simulink library "EngineSystemSubmodel"  (R2014b)
settings: Solver=ode45  StartTime=0.0  StopTime=10.0  FixedStep=1e-4  RelTol=1e-3
values from neighbouring files (symbols this model uses):
  D_turb_wheel = TC.TC_map.turb.D_wheel    [init_MVM.m]
  delta = 2    [Init8RTFLEX68D.m]    (also in Untitled2.m = fcn(p); fcn.m = zeros(size(p)))
  eta_turb_max = TC.TC_map.turb.eff_max    [init_MVM.m]
  flow_coeff_turb = [-1.585326540339;-4.823836967181;1.5853156139822]    [Init8RTFLEX68D.m]    (also in init_MVM.m = TC.TC_map.turb.flow_fit_coeff)
  fs = 0.0683    [Init8RTFLEX68D.m]    (also in NOxProcessGUI.m = varargin{2}; initHybrid.m; initMV.m; init_MVM.m = 0.0682925799315)
  genset = generators(1)    [runTempCyl4S.m]
  J_tc = TC.SAE_map_comp.inertia    [init_MVM.m]
  kai = 1.7    [Init8RTFLEX68D.m]
  Kb = 1*ones(engines,1)    [initHybrid.m]    (also in initMV.m; init_MVM.m = 1; init_ele.m = 1)
  Kd = 20*ones(engines,1)    [initHybrid.m]    (also in initMV.m; init_MVM.m = 10; init_ele.m = 20)
  Ki = 20*ones(engines,1)    [initHybrid.m]    (also in initMV.m; init_MVM.m = 10; init_ele.m = 20)
  Kp = 20*ones(engines,1)    [initHybrid.m]    (also in initMV.m; init_MVM.m = 10; init_ele.m = 20)
  Load_amp = x(4) + xRef(i)    [GetErrGensetResp.m]    (also in runsimulation.m = 0.55; runsimulationRecovery.m = InitialLoad(jj) + LoadStep(ii))
  Load_bias = x(4)    [GetErrGensetResp.m]    (also in runsimulation.m = 0.15; runsimulationRecovery.m = InitialLoad(jj))
  Load_index = 1    [GetErrGensetResp.m]    (also in runsimulation.m; runsimulationRecovery.m)
  N = x*noMol    [NOxProcessGUI.m]    (also in initHybrid.m = .1*ones(engines,1); initMV.m = .1*ones(engines,1); init_ele.m = 0.1)
  omegat0 = RPM_TC_initial/30*pi    [init_MVM.m]
  Start_time = 50    [GetErrGensetResp.m]    (also in runsimulation.m; runsimulationRecovery.m)
  T_load = 1    [GetErrGensetResp.m]    (also in runsimulation.m; runsimulationRecovery.m)
  T_ref_turb = TC.TC_map.turb.T_ref    [init_MVM.m]
  u0 = 0.2    [init_MVM.m]
  Uc_opt = TC.TC_map.turb.Uc_opt    [init_MVM.m]
  uMax = 1.5*ones(engines,1)    [initHybrid.m]    (also in initMV.m; init_MVM.m = 1.1; init_ele.m = 1.1)
  uMin = 0*ones(engines,1)    [initHybrid.m]    (also in initMV.m; init_MVM.m = 0.1; init_ele.m = 0.1)
undefined symbols (not defined in the file or in its folder): CAIPO, control, CV, cyl, eng, engSCont, omega0, rhoG0, Td, Ti, turbo, u_max, volDisp, vSCont, vSDes
undefined symbols (not defined in the file): comp_eff_map, comp_flow_map, n288_rep, npr, nsp, pr_rep, vComp
libraries: EngineSystemSubmodel x167, simulink x2
(part 5 of 5)

== system EngineSystemSubmodel/Flow Restriction/TurbineBus ==
  pTF_u : Inport
  pTF_d : Inport  Port=2
  omegat : Inport  Port=3
  Bus Creator : BusCreator  Inputs=3
  Bus Creator1 : BusCreator  Inputs=3
  Bus Selector : BusSelector  OutputSignals=p,T,F
  Bus Selector1 : BusSelector  OutputSignals=p,T,F
  S-Function : S-Function  FunctionName=turbine_calc_PTF  Parameters=eng.fs,turbo.turb.flowCoeff,turbo.turb.effCoeff  SFunctionModules=GetThdynCombGasZach.c  EnableBusSupport=off
  dmEmb_u : Outport
  dmEmb_d : Outport  Port=2
  Tqt : Outport  Port=3
  Td_calc : Outport  Port=4
  effTurb : Outport  Port=5
  wires:
  S-Function/9 -> effTurb/1
  S-Function/7 -> Tqt/1
  Bus Creator1/1 -> dmEmb_d/1
  Bus Creator/1 -> dmEmb_u/1
  S-Function/3 -> Bus Creator/3  "dmbu"
  S-Function/2 -> Bus Creator/2  "dEu"
  S-Function/1 -> Bus Creator/1  "dmu"
  S-Function/6 -> Bus Creator1/3  "dmbd"
  S-Function/4 -> Bus Creator1/1  "dmd"
  S-Function/5 -> Bus Creator1/2  "dEd"
  S-Function/8 -> Td_calc/1
  pTF_u/1 -> Bus Selector/1
  omegat/1 -> S-Function/7
  pTF_d/1 -> Bus Selector1/1
  Bus Selector1/1 -> S-Function/4  "<p>"
  Bus Selector1/3 -> S-Function/6  "<F>"
  Bus Selector1/2 -> S-Function/5  "<T>"
  Bus Selector/2 -> S-Function/2  "<T>"
  Bus Selector/3 -> S-Function/3  "<F>"
  Bus Selector/1 -> S-Function/1  "<p>"

== system EngineSystemSubmodel/Flow Restriction/TurbineFullMap ==
  pTFu : Inport
  pTFd : Inport  Port=2
  omegaT : Inport  Port=3
  Bus Creator : BusCreator  Inputs=3
  Bus Creator1 : BusCreator  Inputs=3
  Bus Selector2 : BusSelector  OutputSignals=p,T,F
  Bus Selector3 : BusSelector  OutputSignals=p,T,F
  S-Function1 : S-Function  FunctionName=turbine_calc_PTFV1  Parameters=eng.fs,turb.flowMap,turb.effMap,turb.prRep,turb.n298Rep,int32(turb.npr),int32(turb.nsp)  EnableBusSupport=off
  dmEmbu : Outport
  dmEmbd : Outport  Port=2
  tqT : Outport  Port=3
  etaTurb : Outport  Port=4
  Td_calc : Outport  Port=5
  wires:
  Bus Selector2/2 -> S-Function1/2  "<T>"
  Bus Selector3/2 -> S-Function1/5  "<T>"
  S-Function1/3 -> Bus Creator/3  "dmbu"
  Bus Selector2/3 -> S-Function1/3  "<F>"
  S-Function1/6 -> Bus Creator1/3  "dmbd"
  omegaT/1 -> S-Function1/7
  S-Function1/8 -> etaTurb/1  "etaTurb"
  S-Function1/1 -> Bus Creator/1  "dmu"
  pTFu/1 -> Bus Selector2/1
  Bus Selector2/1 -> S-Function1/1  "<p>"
  pTFd/1 -> Bus Selector3/1
  Bus Selector3/1 -> S-Function1/4  "<p>"
  S-Function1/5 -> Bus Creator1/2  "dEd"
  S-Function1/7 -> tqT/1  "tqT"
  Bus Selector3/3 -> S-Function1/6  "<F>"
  S-Function1/2 -> Bus Creator/2  "dEu"
  S-Function1/4 -> Bus Creator1/1  "dmd"
  Bus Creator/1 -> dmEmbu/1
  Bus Creator1/1 -> dmEmbd/1
  S-Function1/9 -> Td_calc/1

== system EngineSystemSubmodel/Flow Restriction/TurbineMV ==
  pTF_u : Inport
  pTF_d : Inport  Port=2
  omegat : Inport  Port=3
  Demux : Demux  Outputs=3
  Demux1 : Demux  Outputs=3
  Mux : Mux  Inputs=3
  Mux1 : Mux  Inputs=3
  S-Function : S-Function  FunctionName=turbine_calc_MV_PTF  Parameters=fs,flow_coeff_turb,D_turb_wheel,Uc_opt,eta_turb_max,T_ref_turb  SFunctionModules=GetThdynCombGasZach.c  EnableBusSupport=off
  dmEmb_u : Outport
  dmEmb_d : Outport  Port=2
  Tqt : Outport  Port=3
  Td_calc : Outport  Port=4
  eta_t : Outport  Port=5
  wires:
  Demux/1 -> S-Function/1
  Demux/3 -> S-Function/3
  Demux/2 -> S-Function/2
  Demux1/2 -> S-Function/5
  Demux1/3 -> S-Function/6
  Demux1/1 -> S-Function/4
  pTF_d/1 -> Demux1/1
  omegat/1 -> S-Function/7
  pTF_u/1 -> Demux/1
  S-Function/8 -> Td_calc/1
  S-Function/5 -> Mux1/2
  S-Function/4 -> Mux1/1
  S-Function/6 -> Mux1/3
  S-Function/1 -> Mux/1
  S-Function/2 -> Mux/2
  S-Function/3 -> Mux/3
  Mux/1 -> dmEmb_u/1
  Mux1/1 -> dmEmb_d/1
  S-Function/7 -> Tqt/1
  S-Function/9 -> eta_t/1

== system EngineSystemSubmodel/Flow Restriction/TurbineMVBus ==
  pTF_u : Inport
  pTF_d : Inport  Port=2
  omegat : Inport  Port=3
  Bus Creator : BusCreator  Inputs=3
  Bus Creator1 : BusCreator  Inputs=3
  Bus Selector : BusSelector  OutputSignals=p,T,F
  Bus Selector1 : BusSelector  OutputSignals=p,T,F
  S-Function : S-Function  FunctionName=turbine_calc_MV_PTF  Parameters=eng.fs,eng.turbo.turb.flowCoeff,eng.turbo.turb.dTurbWheel,eng.turbo.turb.ucOpt,eng.turbo.turb.effMax,eng.turbo.turb.tempRef  SFunctionModules=GetThdynCombGasZach.c  EnableBusSupport=off
  dmEmb_u : Outport
  dmEmb_d : Outport  Port=2
  Tqt : Outport  Port=3
  Td_calc : Outport  Port=4
  eta_t : Outport  Port=5
  wires:
  pTF_u/1 -> Bus Selector/1
  Bus Selector/2 -> S-Function/2  "<T>"
  Bus Selector/3 -> S-Function/3  "<F>"
  Bus Selector/1 -> S-Function/1  "<p>"
  pTF_d/1 -> Bus Selector1/1
  Bus Selector1/2 -> S-Function/5  "<T>"
  Bus Selector1/3 -> S-Function/6  "<F>"
  Bus Selector1/1 -> S-Function/4  "<p>"
  omegat/1 -> S-Function/7
  S-Function/1 -> Bus Creator/1  "dmu"
  S-Function/2 -> Bus Creator/2  "dEu"
  S-Function/3 -> Bus Creator/3  "dmbu"
  Bus Creator/1 -> dmEmb_u/1
  S-Function/4 -> Bus Creator1/1  "dmd"
  S-Function/5 -> Bus Creator1/2  "dEd"
  S-Function/6 -> Bus Creator1/3  "dmbd"
  Bus Creator1/1 -> dmEmb_d/1
  S-Function/7 -> Tqt/1
  S-Function/8 -> Td_calc/1
  S-Function/9 -> eta_t/1

== system EngineSystemSubmodel/Flow Restriction/blower ==
  pTFScav : Inport
  pTFU : Inport  Port=2
  pTFD : Inport  Port=3
  BlowerControl : Subsystem
  Terminator7 : Terminator
  blower1 : S-Function  FunctionName=blower  Parameters=blower.effBlower,blower.coeffBlowerFlow,eng.fs  SFunctionModules=GetThdynCombGasZach  EnableBusSupport=off
  dmEmbU : Outport
  dmEmbD : Outport  Port=2
  wires:
  blower1/2 -> dmEmbD/1  "dmEmbBlower_d"
  blower1/1 -> dmEmbU/1  "dmEmbBlower_u"
  blower1/3 -> Terminator7/1  "powBlower"
  BlowerControl/1(blowerOut) -> blower1/3
  pTFScav/1 -> BlowerControl/1(pTFScav)
  pTFD/1 -> blower1/2
  pTFU/1 -> blower1/1

== system EngineSystemSubmodel/Flow Restriction/blowerFit ==
  pTFScav : Inport
  pTFU : Inport  Port=2
  pTFD : Inport  Port=3
  pScavRef : Inport  Port=4
  BlowerControl : Subsystem  mask{upper=eng.control.blower.upper, lower=eng.control.blower.lower, tauBlower=eng.control.blower.tau}
      mask prompts: upper "Upper bound of scavenge pressure for turning off the blower"; lower "Lower bound of scavenge pressure for turning on the blower"; tauBlower "Time constant for blower starting / stop [s]"
  Demux : Demux  Outputs=3
  Demux1 : Demux  Outputs=3
  PIDControlAntiWinding : EngineSystemSubmodel/Control System/PIDControlAntiWinding  Kp=eng.control.blowerFit.Kp  Td=eng.control.blowerFit.Td  N=eng.control.blowerFit.N  Ti=eng.control.blowerFit.Ti  uMax=eng.control.blowerFit.uMax  uMin=eng.control.blowerFit.uMin  u0=eng.control.blowerFit.u0  Kb=eng.control.blowerFit.Kb
  S-Function : S-Function  FunctionName=blowerFit  Parameters=eng.blower.effBlower,eng.fs  EnableBusSupport=off
  Terminator{,1..5} (6 alike) : Terminator
  engSpeedLPFilterBW4 : S-Function  FunctionName=lowPassFilterBW4  Parameters=BW,y0  EnableBusSupport=off  mask{BW=0.66, y0=1e5}
      mask prompts: BW "Bandwidth [Hz]"; y0 "Initial output"
  dmEmbD : Outport
  dmEmbU : Outport  Port=2
  wires:
  pTFScav/1 -> Demux/1
  S-Function/1 -> Demux1/1, dmEmbU/1  "dmEmbBlower_u"
  S-Function/2 -> dmEmbD/1  "dmEmbBlower_d"
  PIDControlAntiWinding/1 -> PIDControlAntiWinding/3, S-Function/4
  pScavRef/1 -> PIDControlAntiWinding/2
  Demux/1 -> engSpeedLPFilterBW4/1
  Demux/2 -> Terminator/1
  Demux/3 -> Terminator1/1
  pTFU/1 -> S-Function/1
  pTFD/1 -> S-Function/2
  BlowerControl/1(wasteGateOpen) -> S-Function/3
  S-Function/3 -> Terminator2/1  "powBlower"
  Demux1/1 -> Terminator5/1  "dmBlower"
  Demux1/2 -> Terminator3/1
  Demux1/3 -> Terminator4/1
  engSpeedLPFilterBW4/1 -> PIDControlAntiWinding/1, BlowerControl/1(pScav)

== system EngineSystemSubmodel/Gas Exchange/Scavenging ==
  pCyl : Inport
  TCyl : Inport  Port=2
  FCyl : Inport  Port=3
  pIn : Inport  Port=4
  TIn : Inport  Port=5
  FIn : Inport  Port=6
  mDotIn : Inport  Port=7
  combState : Inport  Port=8
  phi : Inport  Port=9
  S-Function1 : S-Function  FunctionName=scavenging1Zone  Parameters=cyl.gasEx.kai,cyl.gasEx.delta,eng.fs,cyl.dim.vDisp,cyl.scavPort.cASPO*180/pi  EnableBusSupport=off
  TOut : Outport
  FOut : Outport  Port=2
  lambdaS : Outport  Port=3
  beta : Outport  Port=4
  wires:
  pCyl/1 -> S-Function1/1
  TCyl/1 -> S-Function1/2
  mDotIn/1 -> S-Function1/7
  TIn/1 -> S-Function1/5
  FCyl/1 -> S-Function1/3
  pIn/1 -> S-Function1/4
  combState/1 -> S-Function1/8
  FIn/1 -> S-Function1/6
  phi/1 -> S-Function1/9
  S-Function1/1 -> TOut/1
  S-Function1/3 -> lambdaS/1
  S-Function1/4 -> beta/1
  S-Function1/2 -> FOut/1

== system EngineSystemSubmodel/Gas Exchange/ScavengingBus ==
  pTFVCyl : Inport
  pTFVIn : Inport  Port=2
  dmEmbIn : Inport  Port=3
  combState : Inport  Port=4
  phi : Inport  Port=5
  Bus Selector : BusSelector  OutputSignals=p,T,F
  Bus Selector1 : BusSelector  OutputSignals=p,T,F
  Bus Selector3 : BusSelector  OutputSignals=dmd
  S-Function : S-Function  FunctionName=scavenging1Zone  Parameters=kai,delta,fs,volDisp,CAIPO*180/pi  EnableBusSupport=off
  TOut : Outport
  FOut : Outport  Port=2
  lambdaS : Outport  Port=3
  beta : Outport  Port=4
  wires:
  pTFVCyl/1 -> Bus Selector/1
  pTFVIn/1 -> Bus Selector1/1
  dmEmbIn/1 -> Bus Selector3/1
  Bus Selector3/1 -> S-Function/7  "<dmd>"
  combState/1 -> S-Function/8
  phi/1 -> S-Function/9
  S-Function/1 -> TOut/1  "T"
  S-Function/3 -> lambdaS/1
  S-Function/4 -> beta/1
  S-Function/2 -> FOut/1  "F"
  Bus Selector/1 -> S-Function/1  "<p>"
  Bus Selector/2 -> S-Function/2  "<T>"
  Bus Selector/3 -> S-Function/3  "<F>"
  Bus Selector1/1 -> S-Function/4  "<p>"
  Bus Selector1/2 -> S-Function/5  "<T>"
  Bus Selector1/3 -> S-Function/6  "<F>"

== system EngineSystemSubmodel/Heat Transfer/EngCylHeatTransfer ==
  pTF_Cyl : Inport
  vCyl : Inport  Port=2
  omega : Inport  Port=3
  Demux : Demux  Outputs=3
  S-Function : S-Function  FunctionName=EngCylHeatTransfer  Parameters=cyl.dim.S,cyl.dim.B,cyl.HT.cAlpha,cyl.HT.mCp,cyl.HT.tempWall0,cyl.HT.cCylHT,eng.nCyl  EnableBusSupport=off
  Terminator : Terminator
  dQ : Outport
  tempWall : Outport  Port=2
  wires:
  S-Function/1 -> dQ/1
  S-Function/2 -> tempWall/1
  pTF_Cyl/1 -> Demux/1
  Demux/1 -> S-Function/1
  Demux/2 -> S-Function/2
  Demux/3 -> Terminator/1
  vCyl/1 -> S-Function/3
  omega/1 -> S-Function/4

== system EngineSystemSubmodel/Heat Transfer/EngCylHeatTransferBus ==
  pTFV_Cyl : Inport
  omega : Inport  Port=2
  Bus Selector : BusSelector  OutputSignals=p,T,V
  S-Function : S-Function  FunctionName=EngCylHeatTransfer  Parameters=cyl.dim.S,cyl.dim.B,cyl.HT.cAlpha,cyl.HT.mCp,cyl.HT.tempWall0,cyl.HT.cCylHT,eng.nCyl  EnableBusSupport=off
  dQ : Outport
  tempWall : Outport  Port=2
  wires:
  S-Function/1 -> dQ/1
  S-Function/2 -> tempWall/1
  pTFV_Cyl/1 -> Bus Selector/1
  omega/1 -> S-Function/4
  Bus Selector/2 -> S-Function/2  "<T>"
  Bus Selector/3 -> S-Function/3  "<V>"
  Bus Selector/1 -> S-Function/1  "<p>"

== system EngineSystemSubmodel/Heat Transfer/EngCylHeatTransferSSTune ==
  pTF_Cyl : Inport
  VCyl : Inport  Port=2
  omega : Inport  Port=3
  tempWall : Inport  Port=4
  Demux : Demux  Outputs=3
  S-Function : S-Function  FunctionName=EngCylHeatTransferSSTune  Parameters=cyl.dim.S,cyl.dim.B,cyl.HT.cAlpha,eng.nCyl  EnableBusSupport=off
  Terminator : Terminator
  dQ : Outport
  wires:
  Demux/1 -> S-Function/1
  Demux/2 -> S-Function/2
  pTF_Cyl/1 -> Demux/1
  omega/1 -> S-Function/4
  S-Function/1 -> dQ/1
  tempWall/1 -> S-Function/5
  Demux/3 -> Terminator/1
  VCyl/1 -> S-Function/3

== system EngineSystemSubmodel/Heat Transfer/EngCylHeatTransferSSTuneBus ==
  pTFV_Cyl : Inport
  omega : Inport  Port=2
  tempWall : Inport  Port=3
  Bus Selector : BusSelector  OutputSignals=p,T,V
  S-Function : S-Function  FunctionName=EngCylHeatTransferSSTune  Parameters=cyl.dim.S,cyl.dim.B,cyl.HT.cAlpha, cyl.HT.cCylHT, eng.nCyl  EnableBusSupport=off
  dQ : Outport
  wires:
  tempWall/1 -> S-Function/5
  S-Function/1 -> dQ/1
  omega/1 -> S-Function/4
  pTFV_Cyl/1 -> Bus Selector/1
  Bus Selector/2 -> S-Function/2  "<T>"
  Bus Selector/3 -> S-Function/3  "<V>"
  Bus Selector/1 -> S-Function/1  "<p>"

== system EngineSystemSubmodel/Load/Load ==
  input : Inport
  Constant : Constant  Value=Load_bias
  Constant2 : Constant  Value=Load_index
  From Workspace : FromWorkspace  VariableName=Tq_hist  SampleTime=0
  Multiport Switch : MultiPortSwitch  Inputs=6
  Ramp : simulink/Sources/Ramp  slope=Load_amp  start=Start_time  X0=Load_bias
  Sine Wave : Sin  Amplitude=Load_amp  Bias=Load_bias  Frequency=2*pi/T_load  SampleTime=0
  Step : Step  Time=Start_time  Before=Load_bias  After=Load_amp  SampleTime=0
  Transport Delay : TransportDelay  DelayTime=Start_time  InitialOutput=Load_bias
  Transport Delay1 : TransportDelay  DelayTime=Start_time  InitialOutput=Load_bias
  Transport Delay2 : TransportDelay  DelayTime=Start_time  InitialOutput=Load_bias
  Out1 : Outport
  wires:
  Constant2/1 -> Multiport Switch/1
  input/1 -> Transport Delay2/1
  Transport Delay/1 -> Multiport Switch/3
  Transport Delay2/1 -> Multiport Switch/6
  Transport Delay1/1 -> Multiport Switch/5
  Step/1 -> Multiport Switch/2
  Sine Wave/1 -> Transport Delay/1
  Multiport Switch/1 -> Out1/1
  Constant/1 -> Multiport Switch/7
  Ramp/1 -> Multiport Switch/4
  From Workspace/1 -> Transport Delay1/1

== system EngineSystemSubmodel/MVEM_TC/TurbochargerShaft ==
  tqComp : Inport
  tqTurb : Inport  Port=2
  Gain1 : Gain
  Gain3 : Gain  Gain=1/genset.eng.jTC
  Integrator : Integrator  InitialCondition=genset.eng.omegaT0*genset.eng.jTC
  Saturation : Saturate  UpperLimit=genset.eng.RPMtMax*pi/30*1.1;  LowerLimit=genset.eng.RPMtMax*pi/30*0.24;
  Sum10 : Sum  Inputs=-+|
  Sum9 : Sum  Inputs=-++
  omegaTC : Outport
  wires:
  Gain1/1 -> Sum9/3
  Saturation/1 -> omegaTC/1, Sum10/2
  Sum10/1 -> Gain1/1
  Gain3/1 -> Sum10/1, Saturation/1  "omegat"
  Integrator/1 -> Gain3/1
  Sum9/1 -> Integrator/1
  tqTurb/1 -> Sum9/2
  tqComp/1 -> Sum9/1

== system EngineSystemSubmodel/Mechanical Part/CrankMechKinematic ==
  pCyl : Inport
  omega : Inport  Port=2
  pScav : Inport  Port=3
  Integrator : Integrator  InitialCondition=cyl.init.phi0rad
  S-Function : S-Function  FunctionName=crankMechKinematic1  Parameters=cyl.dim.B,cyl.dim.S,cyl.dim.lambda  EnableBusSupport=off
  dV : Outport
  Tq : Outport  Port=2
  pow : Outport  Port=3
  phi : Outport  Port=4
  wires:
  pScav/1 -> S-Function/4
  Integrator/1 -> S-Function/3, phi/1
  omega/1 -> Integrator/1, S-Function/2
  pCyl/1 -> S-Function/1
  S-Function/3 -> pow/1
  S-Function/2 -> Tq/1
  S-Function/1 -> dV/1

== system EngineSystemSubmodel/Mechanical Part/Shaft ==
  tqEng : Inport
  tqLoad : Inport  Port=2
  Gain : Gain  Gain=1/eng.jShaft  ParamDataTypeStr=double  OutDataTypeStr=double
  Integrator : Integrator  InitialCondition=eng.jShaft*eng.omegaE0
  MATLAB Function : MATLAB Function  TreatAsAtomicUnit=on  mask{omegaEMax=eng.RPMMax*pi/30, coeffMechEff=eng.coeffMechEff}
      mask prompts: omegaEMax "Maximum engine speed (rad/s)"; coeffMechEff "Coefficient for mechanical efficiency model (2x1)"
  Product : Product
  Sum : Sum  Inputs=|-+
  omegaE : Outport
  TqShaft : Outport  Port=2
  wires:
  tqLoad/1 -> Sum/1
  Integrator/1 -> Gain/1
  tqEng/1 -> Product/1
  MATLAB Function/1(effMech) -> Product/2  "effMech"
  Product/1 -> Sum/2, TqShaft/1  "TqShaft"
  Sum/1 -> Integrator/1
  Gain/1 -> MATLAB Function/1(omegaE), omegaE/1

== system EngineSystemSubmodel/ThermodynamicCalculation/GetXCombGas ==
  note: Output is in mole fraction of the follwoing composition
      |   H;O;N;H2;OH;CO;NO;O2;H2O;CO2;N2;Ar
  pTF : Inport
  Bus Selector : BusSelector  OutputSignals=p,T,F
  S-Function : S-Function  FunctionName=GetXCombGas  Parameters=eng.fs,eng.cyl.comb.T_L,eng.cyl.comb.T_H,eng.cyl.comb.FC,eng.xAir  EnableBusSupport=off
  X : Outport
  wires:
  S-Function/1 -> X/1
  Bus Selector/1 -> S-Function/1  "<p>"
  Bus Selector/2 -> S-Function/2  "<T>"
  Bus Selector/3 -> S-Function/3  "<F>"
  pTF/1 -> Bus Selector/1

== system EngineSystemSubmodel/ThermodynamicCalculation/ThdynCombGasZach ==
  pTF : Inport
  Bus Creator : BusCreator  Inputs=5
  Bus Selector : BusSelector  OutputSignals=p,T,F
  S-Function : S-Function  FunctionName=GetThdynCombGasZachSFunc  Parameters=eng.fs  EnableBusSupport=off
  RhusCp : Outport
  wires:
  Bus Selector/1 -> S-Function/1  "<p>"
  Bus Selector/2 -> S-Function/2  "<T>"
  Bus Selector/3 -> S-Function/3  "<F>"
  pTF/1 -> Bus Selector/1  "p"
  S-Function/3 -> Bus Creator/3  "u"
  S-Function/2 -> Bus Creator/2  "h"
  S-Function/4 -> Bus Creator/4  "s"
  S-Function/5 -> Bus Creator/5  "Cp"
  S-Function/1 -> Bus Creator/1  "R"
  Bus Creator/1 -> RhusCp/1

== system EngineSystemSubmodel/Components/TurbochargerFullModel/Friction ==
  In1 : Inport
  Constant : Constant  Value=turbo.fricCoeff(3)
  Gain1 : Gain  Gain=turbo.fricCoeff(1)
  Gain2 : Gain  Gain=turbo.fricCoeff(2)
  Math Function : Math  Operator=square  SaturateOnIntegerOverflow=on
  Sum1 : Sum  Inputs=+++
  Out1 : Outport
  wires:
  Sum1/1 -> Out1/1
  In1/1 -> Math Function/1, Gain2/1
  Math Function/1 -> Gain1/1
  Gain2/1 -> Sum1/2
  Gain1/1 -> Sum1/1
  Constant/1 -> Sum1/3

== system EngineSystemSubmodel/Components/WasteGate/wasteGateControl ==
  dmExhBypass : Inport
  dmExhTotal : Inport  Port=2
  pScav : Inport  Port=3
  u saturated : Inport  Port=4  PortDimensions=1
  Constant : Constant  Value=1e-6
  Constant1 : Constant  Value=bypassRatio  mask{bypassRatio=bypassRatio}
      mask prompts: bypassRatio "Bypass ratio"
  Gain : Gain  Gain=Kp  mask{Kp=Kp}
      mask prompts: Kp "Proportional gain"
  Gain1 : Gain  Gain=TiInv  mask{Ti=Ti, TiInv=0}
      mask prompts: Ti "Integral time constant"; TiInv "Inverse of time constant"
      mask init:
      | TiInv = 1./Ti;
  Gain2 : Gain  Gain=Kp  mask{Kp=Kp}
      mask prompts: Kp "Proportional gain"
  Gain3 : Gain  Gain=K_b  mask{K_b=K_b}
      mask prompts: K_b "Back calculation gain for anti-windup"
  Integrator : Integrator  InitialCondition=1
  Product : Product  Inputs=*/
  Product1 : Product
  S-Function : S-Function  FunctionName=hysterisis  Parameters=upper,lower  EnableBusSupport=off  mask{upper=upper, lower=lower}
      mask prompts: upper "Upper bound"; lower "Lower bound"
  Saturation : Saturate  UpperLimit=max  LowerLimit=min  mask{max=max, min=min}
      mask prompts: max "Maximum allowable valve opening"; min "Maximum allowable valve opening"
  Sum : Sum  Inputs=|++
  Sum1 : Sum  Inputs=|+-
  Sum2 : Sum  Inputs=|++
  Sum3 : Sum  Inputs=|++
  SumI2 : Sum  DisableCoverage=on  Inputs=-+|
  wasteGateOpen : Outport
  wires:
  S-Function/1 -> Product1/1
  pScav/1 -> S-Function/1
  Gain2/1 -> Gain1/1
  Sum3/1 -> Gain2/1
  Gain3/1 -> Sum3/2
  SumI2/1 -> Gain3/1  "u_sat_error"
  u saturated/1 -> SumI2/2
  Sum2/1 -> SumI2/1, Saturation/1
  Sum1/1 -> Gain/1, Sum3/1
  Gain/1 -> Sum2/1
  Gain1/1 -> Integrator/1
  Integrator/1 -> Sum2/2
  Constant/1 -> Sum/2
  Sum/1 -> Product/2
  Product/1 -> Sum1/2
  Constant1/1 -> Sum1/1
  Saturation/1 -> Product1/2
  Product1/1 -> wasteGateOpen/1
  dmExhBypass/1 -> Product/1
  dmExhTotal/1 -> Sum/1

== system EngineSystemSubmodel/Control System/ECSParamId/EVCControl ==
  pComp : Inport
  pCompRef : Inport  Port=2
  Gain : Gain  Gain=Kp  mask{Kp=Kp}
      mask prompts: Kp "Proportional gain"
  Gain1 : Gain  Gain=1/Ti  mask{Ti=Ti}
      mask prompts: Ti "Integral time constant"
  Integrator : Integrator  InitialCondition=1
  Saturation : Saturate  UpperLimit=max  LowerLimit=min  mask{max=max, min=min}
      mask prompts: max "Maximum allowable output"; min "Minimum allowable output"
  Sum1 : Sum  Inputs=|+-
  Sum2 : Sum  Inputs=|++
  EVCRef : Outport
  wires:
  pCompRef/1 -> Sum1/2  "pCompRef"
  pComp/1 -> Sum1/1  "pComp"
  Sum1/1 -> Gain/1
  Gain/1 -> Gain1/1, Sum2/1
  Gain1/1 -> Integrator/1
  Integrator/1 -> Sum2/2
  Sum2/1 -> Saturation/1
  Saturation/1 -> EVCRef/1

== system EngineSystemSubmodel/Control System/ECSParamId/InjectionControl ==
  deltaPComb : Inport
  deltaPCombRef : Inport  Port=2
  Constant : Constant  Value=Ti  mask{Ti=Ti}
      mask prompts: Ti "Time constant"
  Gain : Gain  Gain=Kp
  Integrator : Integrator  InitialCondition=1
  Product : Product  Inputs=*/
  Saturation : Saturate  UpperLimit=max  LowerLimit=min  mask{max=max, min=min}
      mask prompts: max "Maximum allowable maximum cylinder pressure"; min "Minimum allowable maximum cylinder pressure"
  Sum1 : Sum  Inputs=|+-
  Sum2 : Sum  Inputs=|++
  phiInjRef : Outport
  wires:
  deltaPCombRef/1 -> Sum1/2  "deltaPCombRef"
  deltaPComb/1 -> Sum1/1  "deltaPComb"
  Sum1/1 -> Gain/1
  Gain/1 -> Product/1, Sum2/1
  Product/1 -> Integrator/1
  Integrator/1 -> Sum2/2
  Sum2/1 -> Saturation/1
  Saturation/1 -> phiInjRef/1
  Constant/1 -> Product/2

== system EngineSystemSubmodel/Control System/ECSParamId/maxPCylMaxControl ==
  BSFCMeas : Inport
  BSFCRef : Inport  Port=2
  Constant : Constant  Value=Ti  mask{Ti=Ti}
      mask prompts: Ti "Time constant"
  Gain : Gain  Gain=Kp
  Integrator : Integrator  InitialCondition=100
  Product : Product  Inputs=*/
  Saturation : Saturate  UpperLimit=max  LowerLimit=min
  Sum1 : Sum  Inputs=|+-
  Sum2 : Sum  Inputs=|++
  pMaxRef : Outport
  wires:
  BSFCRef/1 -> Sum1/2  "BSFCRef"
  BSFCMeas/1 -> Sum1/1  "BSFCMeas"
  Sum1/1 -> Gain/1
  Gain/1 -> Product/1, Sum2/1
  Product/1 -> Integrator/1
  Integrator/1 -> Sum2/2
  Sum2/1 -> Saturation/1
  Saturation/1 -> pMaxRef/1
  Constant/1 -> Product/2

== system EngineSystemSubmodel/Control System/ECSParamId/tempWallControl ==
  dQCyl : Inport
  dQCylRef : Inport  Port=2
  Constant : Constant  Value=Ti  mask{Ti=Ti}
      mask prompts: Ti "Time constant"
  Constant1 : Constant  Value=swTWCont
  Gain : Gain  Gain=Kp
  Integrator : Integrator  InitialCondition=700
  Product : Product  Inputs=*/
  Product1 : Product  Inputs=**
  Sum1 : Sum  Inputs=|+-
  Sum2 : Sum  Inputs=|++
  TWall : Outport
  wires:
  dQCyl/1 -> Sum1/1  "QCyl"
  Sum1/1 -> Gain/1
  Gain/1 -> Product/1, Sum2/1
  Product/1 -> Integrator/1
  Integrator/1 -> Sum2/2
  Product1/1 -> TWall/1
  Constant/1 -> Product/2
  dQCylRef/1 -> Sum1/2
  Sum2/1 -> Product1/2
  Constant1/1 -> Product1/1

== system EngineSystemSubmodel/Control System/Governor/PID controller ==
  e : Inport  PortDimensions=1
  omega_pu : Inport  Port=2  PortDimensions=1
  u saturated : Inport  Port=3  PortDimensions=1
  D : Gain  DisableCoverage=on  Gain=genset.governor.N
  Filter : Integrator  DisableCoverage=on  InitialCondition=-genset.omega0*genset.governor.Kd
  Gain2 : Gain  Gain=-genset.governor.Kd
  I : Gain  Gain=genset.governor.Ki
  Integrator : Integrator  DisableCoverage=on  InitialCondition=genset.u0
  Kb : Gain  DisableCoverage=on  Gain=genset.governor.Kb  ParamDataTypeStr=Inherit: Inherit from 'Gain'
  P : Gain  Gain=genset.governor.Kp
  Saturation : Saturate  UpperLimit=genset.u_max  LowerLimit=genset.u_min  LinearizeAsGain=off  OutMin=genset.u_min  OutMax=genset.u_max  OutDataTypeStr=Inherit: Inherit via back propagation
  Sum1 : Sum  Inputs=+++
  SumD : Sum  DisableCoverage=on  Inputs=|+-
  SumI1 : Sum  DisableCoverage=on  Inputs=|++
  SumI2 : Sum  DisableCoverage=on  Inputs=-+|
  u : Outport  PortDimensions=1  InitialOutput=0
  wires:
  I/1 -> Integrator/1
  SumI1/1 -> I/1
  u saturated/1 -> SumI2/2
  Kb/1 -> SumI1/2
  SumI2/1 -> Kb/1  "u_sat_error"
  Sum1/1 -> SumI2/1, Saturation/1
  Gain2/1 -> SumD/1
  SumD/1 -> D/1
  Filter/1 -> SumD/2  "xid"
  Saturation/1 -> u/1
  P/1 -> Sum1/1  "governor_P"
  e/1 -> SumI1/1, P/1  "err_governor"
  omega_pu/1 -> Gain2/1
  D/1 -> Filter/1, Sum1/2  "governor_D"
  Integrator/1 -> Sum1/3  "governor_I"

== system EngineSystemSubmodel/Control System/Governor_SpeedControl/PID controller ==
  e : Inport  PortDimensions=1
  omega_pu : Inport  Port=2  PortDimensions=1
  u saturated : Inport  Port=3  PortDimensions=1
  D : Gain  DisableCoverage=on  Gain=N
  Filter : Integrator  DisableCoverage=on  InitialCondition=-omega0*Kd
  Gain2 : Gain  Gain=Kd
  I : Gain  Gain=Ki
  Integrator : Integrator  DisableCoverage=on  InitialCondition=u0
  Kb : Gain  DisableCoverage=on  Gain=Kb  ParamDataTypeStr=Inherit: Inherit from 'Gain'
  P : Gain  Gain=Kp
  Saturation : Saturate  UpperLimit=u_max  LowerLimit=u_min  LinearizeAsGain=off  OutMin=u_min  OutMax=u_max  OutDataTypeStr=Inherit: Inherit via back propagation
  Sum1 : Sum  Inputs=+++
  SumD : Sum  DisableCoverage=on  Inputs=|+-
  SumI1 : Sum  DisableCoverage=on  Inputs=|++
  SumI2 : Sum  DisableCoverage=on  Inputs=-+|
  u : Outport  PortDimensions=1  InitialOutput=0
  wires:
  I/1 -> Integrator/1
  SumI1/1 -> I/1
  u saturated/1 -> SumI2/2
  Kb/1 -> SumI1/2
  SumI2/1 -> Kb/1  "u_sat_error"
  Sum1/1 -> SumI2/1, Saturation/1
  Gain2/1 -> SumD/1
  SumD/1 -> D/1
  Filter/1 -> SumD/2  "xid"
  Saturation/1 -> u/1
  P/1 -> Sum1/1  "governor_P"
  e/1 -> SumI1/1, P/1
  omega_pu/1 -> Gain2/1
  D/1 -> Filter/1, Sum1/2  "governor_D"
  Integrator/1 -> Sum1/3  "governor_I"

== system EngineSystemSubmodel/Control System/Smoke Limiter/LP_T0_2 ==
  In1 : Inport
  Gain3 : Gain  Gain=100
  Integrator : Integrator  InitialCondition=1
  Sum : Sum  Inputs=|+-
  Out1 : Outport
  wires:
  Integrator/1 -> Sum/2, Out1/1
  In1/1 -> Sum/1
  Sum/1 -> Gain3/1
  Gain3/1 -> Integrator/1

== system EngineSystemSubmodel/Control System/Smoke Limiter MV/LP_T0_01 ==
  In1 : Inport
  Gain3 : Gain  Gain=100
  Integrator : Integrator  InitialCondition=1
  Sum : Sum  Inputs=|+-
  Out1 : Outport
  wires:
  Integrator/1 -> Sum/2, Out1/1
  In1/1 -> Sum/1
  Sum/1 -> Gain3/1
  Gain3/1 -> Integrator/1

== system EngineSystemSubmodel/Control System/Smoke Limiter MV/LP_T0_1 ==
  In1 : Inport
  Gain3 : Gain  Gain=100
  Integrator : Integrator  InitialCondition=1
  Sum : Sum  Inputs=|+-
  Out1 : Outport
  wires:
  Integrator/1 -> Sum/2, Out1/1
  In1/1 -> Sum/1
  Sum/1 -> Gain3/1
  Gain3/1 -> Integrator/1

== system EngineSystemSubmodel/Control System/Smoke Limiter MV/LP_T0_2 ==
  In1 : Inport
  Gain3 : Gain  Gain=100
  Integrator : Integrator  InitialCondition=1
  Sum : Sum  Inputs=|+-
  Out1 : Outport
  wires:
  Integrator/1 -> Sum/2, Out1/1
  In1/1 -> Sum/1
  Sum/1 -> Gain3/1
  Gain3/1 -> Integrator/1

== system EngineSystemSubmodel/EngineOperatingParameterCalculation/volEffCalc/MovingAvg ==
  in : Inport
  Gain4 : Gain  Gain=1/TdMA
  Integrator : Integrator  InitialCondition=y0*TdMA
  Sum9 : Sum  Inputs=|+-
  Transport Delay : TransportDelay  DelayTime=TdMA
  Out : Outport
  wires:
  Integrator/1 -> Gain4/1
  in/1 -> Transport Delay/1, Sum9/1
  Transport Delay/1 -> Sum9/2
  Sum9/1 -> Integrator/1
  Gain4/1 -> Out/1

== system EngineSystemSubmodel/EngineOperatingParameterCalculation/volEffCalc/MovingAvg1 ==
  in : Inport
  Gain4 : Gain  Gain=1/TdMA
  Integrator : Integrator  InitialCondition=y0*TdMA
  Sum9 : Sum  Inputs=|+-
  Transport Delay : TransportDelay  DelayTime=TdMA
  Out : Outport
  wires:
  Integrator/1 -> Gain4/1
  in/1 -> Transport Delay/1, Sum9/1
  Transport Delay/1 -> Sum9/2
  Sum9/1 -> Integrator/1
  Gain4/1 -> Out/1

== system EngineSystemSubmodel/Flow Restriction/blower/BlowerControl ==
  pTFScav : Inport
  Abs : Abs
  Constant : Constant
  Demux : Demux  Outputs=3
  S-Function : S-Function  FunctionName=hysterisis  Parameters=upper,lower  EnableBusSupport=off  mask{upper=eng.control.blower.upper, lower=eng.control.blower.lower}
      mask prompts: upper "Upper bound"; lower "Lower bound"
  Subtract : Sum  Inputs=+-
  Terminator : Terminator
  Terminator1 : Terminator
  Transfer Fcn : TransferFcn  Denominator=[eng.control.blower.tau 1]
  blowerOut : Outport
  wires:
  Transfer Fcn/1 -> blowerOut/1
  pTFScav/1 -> Demux/1
  Demux/1 -> S-Function/1  "pScav"
  Demux/2 -> Terminator/1
  Demux/3 -> Terminator1/1
  S-Function/1 -> Subtract/1
  Constant/1 -> Subtract/2
  Subtract/1 -> Abs/1
  Abs/1 -> Transfer Fcn/1

== system EngineSystemSubmodel/Flow Restriction/blowerFit/BlowerControl ==
  pScav : Inport
  S-Function : S-Function  FunctionName=hysterisis  Parameters=upper,lower  EnableBusSupport=off  mask{upper=upper, lower=lower}
      mask prompts: upper "Upper bound"; lower "Lower bound"
  Transfer Fcn : TransferFcn  Denominator=[tauBlower 1]
  wasteGateOpen : Outport
  wires:
  S-Function/1 -> Transfer Fcn/1
  pScav/1 -> S-Function/1  "pScav"
  Transfer Fcn/1 -> wasteGateOpen/1

== matlab function EngineSystemSubmodel/Load/Propeller ==
  data: omegaE input; Tq output; coeffProp parameter
function Tq = propellerLaw(omegaE,coeffProp)
%#codegen
    Tq = ((coeffProp(1)*omegaE + coeffProp(2))*omegaE + coeffProp(3))*1000;
end

== matlab function EngineSystemSubmodel/Components/ControlValve/MATLAB Function ==
  data: u input; x parameter; y parameter; y1 output
function y1 = fcn(u,x,y)
%#codegen
y1 = interp1(x,y,u,'pchip');

== matlab function EngineSystemSubmodel/Mechanical Part/Shaft/MATLAB Function ==
  data: omegaE input; effMech output; omegaEMax parameter; coeffMechEff parameter
function effMech = mechEff(omegaE,omegaEMax,coeffMechEff)
%#codegen
	omega_nom = omegaE/omegaEMax;		
	effMech = 1 - (coeffMechEff(2)*omega_nom - (coeffMechEff(1)/ ...
        (1-coeffMechEff(2)))*(omega_nom-coeffMechEff(2))*omega_nom);
end
